simulink model "abslut50_fixpt20_32"  (R2021b)
settings: Solver=VariableStepAuto  StartTime=0.0  StopTime=99  RelTol=1e-3
undefined symbols (not defined in the file or in its folder): figd2104, xcu250
libraries: hdlBasic x5226, vmcUtilities x1
(part 17 of 17)

== matlab function abslut50_fixpt20_32/MATLAB Function3 ==
  data: u20 input; u21 input; u22 input; u23 input; u24 input; u25 input; u26 input; u27 input; u28 input; u29 input; u30 input; u31 input; u32 input; x input; y20 output; y21 output; y22 output; y23 output; y24 output; y25 output; y26 output; y27 output; y28 output; y29 output; y30 output; y31 output; y32 output
function [y20,y21,y22,y23,y24,y25,y26,y27,y28,y29,y30,y31,y32] = fcn(u20,u21,u22,u23,u24,u25,u26,u27,u28,u29,u30,u31,u32,x)
y20 = (u20 - x).^2;
y21 = (u21 - x).^2;
y22 = (u22 - x).^2;
y23 = (u23 - x).^2;
y24 = (u24 - x).^2;
y25 = (u25 - x).^2;
y26 = (u26 - x).^2;
y27 = (u27 - x).^2;
y28 = (u28 - x).^2;
y29 = (u29 - x).^2;
y30 = (u30 - x).^2;
y31 = (u31 - x).^2;
y32 = (u32 - x).^2;
